simulink model "ThreeTank_NonLinear"  (R2017b)
settings: Solver=VariableStepAuto  StartTime=0.0  StopTime=5000  FixedStep=0.1  RelTol=1e-3
undefined symbols (not defined in the file or in its folder): A1, A2, A3, c0, c1, c2, k, simSwitch, x0
settings Model: Creator=lasse  LastModifiedBy=lasse
settings DataIOCC: ExternalInput=ds  InitialState=x0  SaveFinalState=on  SaveFormat=Array  SaveState=on  TimeSaveName=t

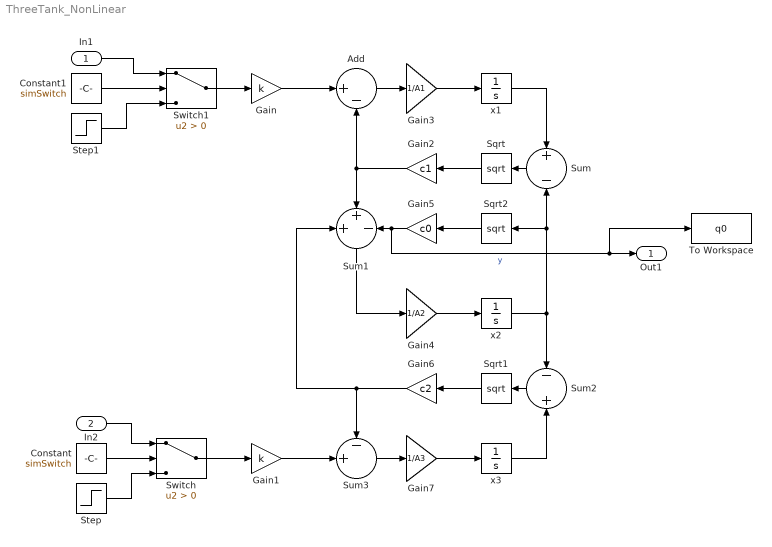
== system ThreeTank_NonLinear ==
  In1 : Inport
  In2 : Inport  Port=2
  Add : Sum  Inputs=|+-
  Constant : Constant  Value=simSwitch
  Constant1 : Constant  Value=simSwitch
  Gain : Gain  Gain=k
  Gain1 : Gain  Gain=k
  Gain2 : Gain  Gain=c1
  Gain3 : Gain  Gain=1/A1
  Gain4 : Gain  Gain=1/A2
  Gain5 : Gain  Gain=c0
  Gain6 : Gain  Gain=c2
  Gain7 : Gain  Gain=1/A3
  Sqrt : Sqrt  SaturateOnIntegerOverflow=on
  Sqrt1 : Sqrt  SaturateOnIntegerOverflow=on
  Sqrt2 : Sqrt  OutputSignalType=real  SaturateOnIntegerOverflow=on
  Step : Step  After=u(2)  SampleTime=0
  Step1 : Step  After=u(1)  SampleTime=0
  Sum : Sum  Inputs=+|-
  Sum1 : Sum  Inputs=++-
  Sum2 : Sum  Inputs=-|+
  Sum3 : Sum  Inputs=-+|
  Switch : Switch  Criteria=u2 > Threshold
  Switch1 : Switch  Criteria=u2 > Threshold
  To Workspace : ToWorkspace  VariableName=q0  SaveFormat=Structure With Time  SampleTime=-1
  x1 : Integrator  Priority=1  InitialCondition=x0(1)
  x2 : Integrator  Priority=2  InitialCondition=x0(2)
  x3 : Integrator  Priority=3  InitialCondition=x0(3)
  Out1 : Outport
  wires:
  Gain/1 -> Add/1
  Gain2/1 -> Sum1/2, Add/2
  Add/1 -> Gain3/1
  Gain3/1 -> x1/1
  x1/1 -> Sum/1
  Gain5/1 -> To Workspace/1, Out1/1, Sum1/3  "y"
  x3/1 -> Sum2/2
  Sum2/1 -> Sqrt1/1
  Sum3/1 -> Gain7/1
  Gain1/1 -> Sum3/2
  Gain4/1 -> x2/1
  Sum1/1 -> Gain4/1
  Gain7/1 -> x3/1
  Gain6/1 -> Sum1/1, Sum3/1
  Sqrt1/1 -> Gain6/1
  Sum/1 -> Sqrt/1
  Sqrt2/1 -> Gain5/1
  Sqrt/1 -> Gain2/1
  Switch/1 -> Gain1/1
  x2/1 -> Sum2/1, Sqrt2/1, Sum/2
  Step/1 -> Switch/3
  In2/1 -> Switch/1
  In1/1 -> Switch1/1
  Step1/1 -> Switch1/3
  Constant1/1 -> Switch1/2
  Switch1/1 -> Gain/1
  Constant/1 -> Switch/2
